simulink library "soccerRobotLib"  (R2019a)
settings: Solver=VariableStepAuto  StartTime=0.0  StopTime=10.0  RelTol=1e-3
values from neighbouring files (symbols this model uses):
  initialPoses = initialPoses + randn(size(initialPoses)).*[3 3 pi/4]    [randomizeStartingPositions.m]
undefined symbols (not defined in the file or in its folder): ballCarryFactor, objDetectorMaxHits, robotColors, robotDetectorMaxHits, sampleTime
libraries: mobileRoboticsLib x4, simulink x1
settings Model: Creator=scastro  LastModifiedBy=scastro
settings DataIOCC: ReturnWorkspaceOutputs=off
settings DebuggingCC: ArithmeticOperatorsInVariantConditions=warning

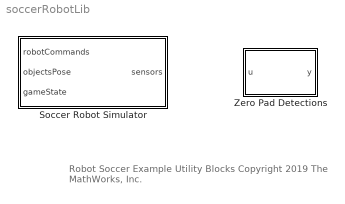
== system soccerRobotLib ==
  note: Robot Soccer Example
      | Utility Blocks
      |
      | Copyright 2019 The MathWorks, Inc.
  Soccer Robot Simulator : Subsystem  mask(Soccer Robot Simulation){robotIdx=1}
      mask prompts: robotIdx "Robot Index"
      mask help: Simulates a soccer robot with object detector
  Zero Pad Detections : MATLAB Function  TreatAsAtomicUnit=on  mask(Zero Pad Detections){maxHits=5}
      mask prompts: maxHits "Maximum Sensor Hits"
      mask help: Zero pads detections matrix so it is fixed-size and works with arrays of buses.

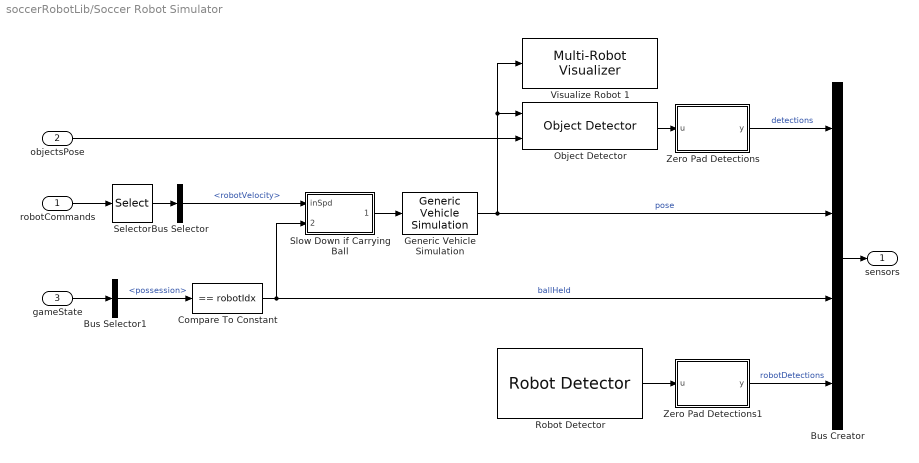
== system soccerRobotLib/Soccer Robot Simulator ==
  robotCommands : Inport
  objectsPose : Inport  Port=2
  gameState : Inport  Port=3
  Bus Creator : BusCreator  Inputs=4  OutDataTypeStr=Bus: RobotSensorBus  NonVirtualBus=on
      settings: InheritFromInputs=off
  Bus Selector : BusSelector  OutputSignals=robotVelocity
  Bus Selector1 : BusSelector  OutputSignals=possession
  Compare To Constant : simulink/Logic and Bit Operations/Compare To Constant  relop===  const=robotIdx  OutDataTypeStr=boolean
  Generic Vehicle Simulation : mobileRoboticsLib/Utilities/Generic Vehicle Simulation  initX=initialPoses(robotIdx,1)  initY=initialPoses(robotIdx,2)  initAngle=initialPoses(robotIdx,3)  Ts=sampleTime
      settings: SourceProductName=Mobile Robotics Simulation Toolbox
  Object Detector : mobileRoboticsLib/Environments/Object Detector  mapName=map  sensorOffset=objDetectorOffset  sensorAngle=objDetectorAngle  fieldOfView=objDetectorFOV  maxRange=objDetectorRange  maxDetections=objDetectorMaxHits  sampleTime=sampleTime
      settings: SourceProductName=Mobile Robotics Simulation Toolbox
  Robot Detector : mobileRoboticsLib/Environments/Robot Detector  robotIdx=robotIdx  sensorOffset=robotDetectorOffset  sensorAngle=robotDetectorAngle  sensorFOV=pi/3  maxRange=robotDetectorRange  maxDetections=robotDetectorMaxHits  sampleTime=sampleTime
      settings: SourceProductName=Mobile Robotics Simulation Toolbox
  Selector : Selector  InputPortWidth=numRobots  IndexOptions=Index vector (dialog)  Indices=robotIdx  OutputSizes=1
  Slow Down if Carrying Ball : Subsystem
  Visualize Robot 1 : mobileRoboticsLib/Environments/Multi-Robot Visualizer  idx=robotIdx  radius=robotRadius  robotColor=robotColors(robotIdx,:)  showTraj=off  hasLidar=off  sensorOffset=[0 0]  scanAngles=0  maxNumScans=0  hasObjDetector=on  objDetectorOffset=objDetectorOffset  objDetectorAngle=objDetectorAngle  objDetectorFOV=objDetectorFOV  objDetectorMaxRange=objDetectorRange  hasRobotDetector=off  robotDetectorOffset=[0,0]  robotDetectorAngle=0  robotDetectorFOV=pi/3  robotDetectorMaxRange=5  robotDetectorNumDetections=0
      settings: SourceProductName=Mobile Robotics Simulation Toolbox
  Zero Pad Detections : MATLAB Function  TreatAsAtomicUnit=on  mask(Zero Pad Detections){maxHits=objDetectorMaxHits}
      mask prompts: maxHits "Maximum Sensor Hits"
      mask help: Zero pads detections matrix so it is fixed-size and works with arrays of buses.
  Zero Pad Detections1 : MATLAB Function  TreatAsAtomicUnit=on  mask(Zero Pad Detections){maxHits=robotDetectorMaxHits}
      mask prompts: maxHits "Maximum Sensor Hits"
      mask help: Zero pads detections matrix so it is fixed-size and works with arrays of buses.
  sensors : Outport
  wires:
  Compare To Constant/1 -> Slow Down if Carrying Ball/2(ballHeld), Bus Creator/3  "ballHeld"
  Bus Selector1/1 -> Compare To Constant/1  "<possession>"
  gameState/1 -> Bus Selector1/1
  Generic Vehicle Simulation/1 -> Object Detector/1, Visualize Robot 1/1, Bus Creator/2  "pose"
  robotCommands/1 -> Selector/1
  Object Detector/1 -> Zero Pad Detections/1(u)
  objectsPose/1 -> Object Detector/2
  Selector/1 -> Bus Selector/1
  Bus Selector/1 -> Slow Down if Carrying Ball/1(inSpd)  "<robotVelocity>"
  Zero Pad Detections/1(y) -> Bus Creator/1  "detections"
  Bus Creator/1 -> sensors/1
  Robot Detector/1 -> Zero Pad Detections1/1(u)
  Zero Pad Detections1/1(y) -> Bus Creator/4  "robotDetections"
  Slow Down if Carrying Ball/1(outSpd) -> Generic Vehicle Simulation/1

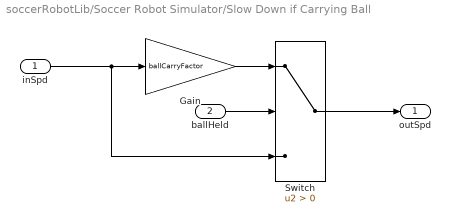
== system soccerRobotLib/Soccer Robot Simulator/Slow Down if Carrying Ball ==
  inSpd : Inport
  ballHeld : Inport  Port=2
  Gain : Gain  Gain=ballCarryFactor
  Switch : Switch  Criteria=u2 > Threshold
  outSpd : Outport
  wires:
  Switch/1 -> outSpd/1
  ballHeld/1 -> Switch/2
  inSpd/1 -> Switch/3, Gain/1
  Gain/1 -> Switch/1

== matlab function soccerRobotLib/Soccer Robot Simulator/Zero Pad Detections ==
  data: u input size=[maxHits 3]; y output size=[maxHits 3]; maxHits parameter
function y = zeroPad(u,maxHits)
% Zero-pads object detections to work with arrays of buses

y = zeros(maxHits,3);
numElems = min(size(u,1),maxHits);
for idx = 1:numElems
   y(idx,1:3) = u(idx,1:3); 
end

== matlab function soccerRobotLib/Zero Pad Detections ==
  data: u input size=[maxHits 3]; y output size=[maxHits 3]; maxHits parameter
function y = zeroPad(u,maxHits)
% Zero-pads object detections to work with arrays of buses

y = zeros(maxHits,3);
numElems = min(size(u,1),maxHits);
for idx = 1:numElems
   y(idx,1:3) = u(idx,1:3); 
end

== matlab function soccerRobotLib/Soccer Robot Simulator/Zero Pad Detections1 ==
  data: u input size=[maxHits 3]; y output size=[maxHits 3]; maxHits parameter
function y = zeroPad(u,maxHits)
% Zero-pads object detections to work with arrays of buses

y = zeros(maxHits,3);
numElems = min(size(u,1),maxHits);
for idx = 1:numElems
   y(idx,1:3) = u(idx,1:3); 
end
